simulink model "Simulink_control"  (R2020b)
settings: Solver=VariableStepAuto  StartTime=0.0  StopTime=inf  RelTol=1e-3
undefined symbols (not defined in the file or in its folder): Angular, Linear
libraries: robotlib x4, robotcorelib x1
settings Model: Creator=brayan  LastModifiedBy=brayan

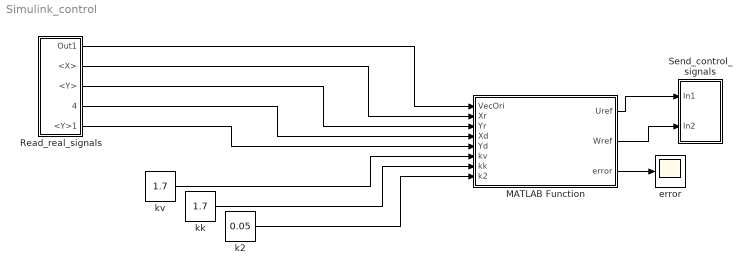
== system Simulink_control ==
  MATLAB Function : MATLAB Function  TreatAsAtomicUnit=on
  Read_real_signals : Subsystem
  Send_control_signals : Subsystem
  error : Scope
  k2 : Constant  Value=0.05
  kk : Constant  Value=1.7
  kv : Constant  Value=1.7
  wires:
  MATLAB Function/3(error) -> error/1
  kv/1 -> MATLAB Function/6(kv)
  kk/1 -> MATLAB Function/7(kk)
  k2/1 -> MATLAB Function/8(k2)
  MATLAB Function/1(Uref) -> Send_control_signals/1(In1)
  MATLAB Function/2(Wref) -> Send_control_signals/2(In2)
  Read_real_signals/1(Out1) -> MATLAB Function/1(VecOri)
  Read_real_signals/2(<X>) -> MATLAB Function/2(Xr)
  Read_real_signals/3(<Y>) -> MATLAB Function/3(Yr)
  Read_real_signals/4(<X>1) -> MATLAB Function/4(Xd)
  Read_real_signals/5(<Y>1) -> MATLAB Function/5(Yd)

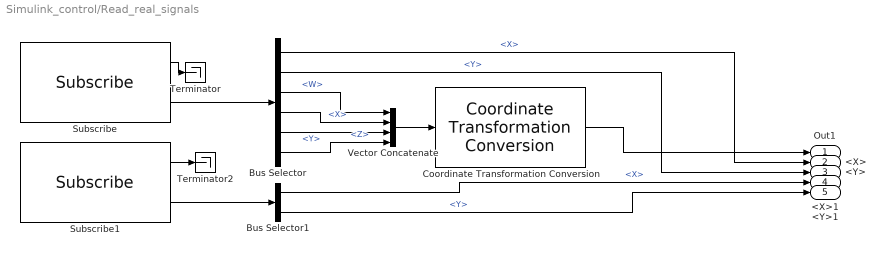
== system Simulink_control/Read_real_signals ==
  Bus Selector : BusSelector  OutputSignals=Pose.Pose.Position.X,Pose.Pose.Position.Y,Pose.Pose.Orientation.W,Pose.Pose.Orientation.X,Pose.Pose.Orientation.Y,Pose.Pose.Orientation.Z
  Bus Selector1 : BusSelector  OutputSignals=Pose.Position.X,Pose.Position.Y
  Coordinate Transformation Conversion : robotcorelib/Coordinate Transformation Conversion  InputRepresentation=Quaternion  InputEulerSequence=ZYX  ShowTrVecInputPort=on  OutputRepresentation=Euler Angles  OutputEulerSequence=ZYX  ShowTrVecOutputPort=on  SimulateUsing=Interpreted execution
      settings: SourceProductBaseCode=NV,RO,RR,UV
  Subscribe : robotlib/Subscribe  topicSource=Select from ROS network  topic=/wamv/sensors/position/p3d_wamv  messageType=nav_msgs/Odometry  SampleTime=-1  legacyBusStruct=off  messageQueueLength=1
  Subscribe1 : robotlib/Subscribe  topicSource=Select from ROS network  topic=/boat/pose_d  messageType=geometry_msgs/PoseStamped  SampleTime=-1  legacyBusStruct=off  messageQueueLength=1
  Terminator : Terminator
  Terminator2 : Terminator
  Vector Concatenate : Concatenate  NumInputs=4
  Out1 : Outport
  <X> : Outport  Port=2
  <Y> : Outport  Port=3
  <X>1 : Outport  Port=4
  <Y>1 : Outport  Port=5
  wires:
  Subscribe/2 -> Bus Selector/1
  Subscribe1/2 -> Bus Selector1/1
  Bus Selector1/1 -> <X>1/1  "<X>"
  Bus Selector/5 -> Vector Concatenate/3  "<Y>"
  Vector Concatenate/1 -> Coordinate Transformation Conversion/1
  Bus Selector/4 -> Vector Concatenate/2  "<X>"
  Subscribe/1 -> Terminator/1
  Bus Selector1/2 -> <Y>1/1  "<Y>"
  Bus Selector/1 -> <X>/1  "<X>"
  Bus Selector/2 -> <Y>/1  "<Y>"
  Bus Selector/6 -> Vector Concatenate/4  "<Z>"
  Coordinate Transformation Conversion/1 -> Out1/1
  Bus Selector/3 -> Vector Concatenate/1  "<W>"
  Subscribe1/1 -> Terminator2/1

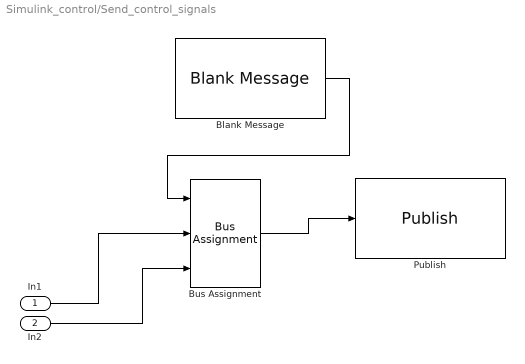
== system Simulink_control/Send_control_signals ==
  In1 : Inport
  In2 : Inport  Port=2
  Blank Message : robotlib/Blank Message  messageClass=Message  entityType=geometry_msgs/Twist  messageType=geometry_msgs/Twist  SampleTime=inf  legacyBusStruct=off
  Bus Assignment : BusAssignment  AssignedSignals=Linear.X,Angular.Z
  Publish : robotlib/Publish  topicSource=Select from ROS network  topic=/boat/cmd  messageType=geometry_msgs/Twist  legacyBusStruct=off  messageQueueLength=1
  wires:
  Bus Assignment/1 -> Publish/1
  Blank Message/1 -> Bus Assignment/1
  In1/1 -> Bus Assignment/2
  In2/1 -> Bus Assignment/3

== matlab function Simulink_control/MATLAB Function ==
  data: VecOri input; Uref output; Xr input; Yr input; Xd input; Yd input; Wref output; error output; kv input; kk input; k2 input
function [Uref, Wref, error] = fcn(VecOri, Xr, Yr, Xd, Yd, kv, kk, k2)
    Xe = Xd - Xr;
    Ye = Yd - Yr;
    error = sqrt(Xe^2 + Ye^2);
    a_e = atan2(Ye, Xe);
    angular_difference=normalangulo(normalangulo(a_e)-normalangulo(VecOri(1)));
    if error <= 0.5
        Uref = 0;
        Wref = 0;          
    else
        Uref = kv * tanh(k2 * error) * cos(angular_difference);
        Wref = kk * angular_difference + kv * (tanh(k2 * error) / error) * sin(angular_difference) * cos(angular_difference);
    end
end

function n_angulo=normalangulo(angulo)
  if angulo > pi
        angulo = angulo - 2*pi;
    elseif angulo < -pi
        angulo = angulo + 2*pi;
    else
        % No se necesita hacer nada
  end
    n_angulo=angulo;
end
